simulink model "hil_fuel_cell_valve"  (R2022a)
settings: Solver=FixedStepDiscrete  StartTime=0.0  StopTime=inf  FixedStep=0.01  RelTol=1e-3  AbsTol=1e-3  EnableMultiTasking=on
model workspace: external: MATLAB File model_workspace.m (data not in the file)
values from neighbouring files (symbols this model uses):
  anode_tube_D = 0.004    [model_workspace.m]
  cathode_tube_D = 0.004    [model_workspace.m]
  env_p = 0.101325    [model_workspace.m]
  env_T = 60    [model_workspace.m]
  N2_T = [-56.55 -50 -40 -30 -20 -10 -5 -4 -3 -2 -1 0 1 2 3 4 5 10 20 30          40 50 60 70 80 90 100 110 120 130 140 150 160 170 180 190 200 210          220 230 240 250 260 270 280 290 300 310 320 330 340 350]    [model_workspace.m]
  radiator_air_area_fins = 11.5625    [model_workspace.m]
  radiator_air_area_primary = 1.2231250000000002    (= 1.223125)    [model_workspace.m]
  radiator_eta_fin = 0.7    [model_workspace.m]
  radiator_rho = 2700    [model_workspace.m]
  radiator_t_wall = 0.0001    [model_workspace.m]
  stack_area = 49    [model_workspace.m]
  stack_iL = 1.4    [model_workspace.m]
  stack_mea_rho = 1800    [model_workspace.m]
  stack_num_cells = 8    [model_workspace.m]
  stack_num_channels = 1    [model_workspace.m]
  stack_t_gdl = 250    [model_workspace.m]
  stack_t_membrane = 125    [model_workspace.m]
  stack_w_channels = 0.4    [model_workspace.m]
  time_step = 0.02    [model_workspace.m]
libraries: fl_lib x102, nesl_utility x42, simulink x7, slpidlib x3
(part 3 of 3)

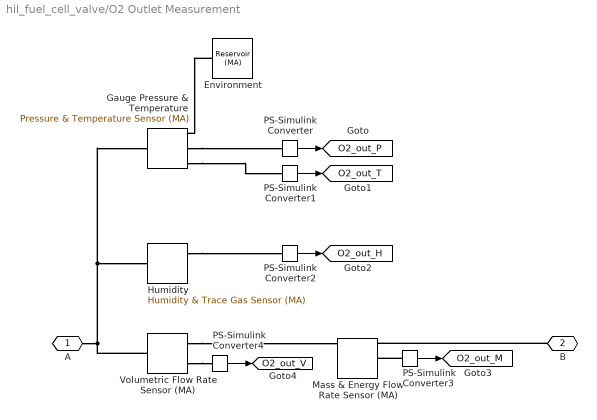
== system hil_fuel_cell_valve/O2 Outlet Measurement ==
  Environment : fl_lib/Moist Air/Elements/Reservoir (MA)  pressure_spec=foundation.enum.pressure_spec.specified  reservoir_pressure=env_p MPa  temperature_spec=foundation.enum.temperature_spec.specified  reservoir_temperature=env_T degC  moisture_spec=foundation.enum.moisture_spec.relative_humidity  reservoir_RH=0  reservoir_x_w=0.01  reservoir_y_w=0.01  reservoir_HR=0.01  trace_gas_spec=foundation.enum.trace_gas_spec.mole_fraction  reservoir_x_g=0.001  reservoir_y_g=tank_yH2  RH_ws=1  area_A=pi*anode_tube_D^2/4 m^2
      settings: SourceProductBaseCode=PW,SS,VE
  Gauge Pressure & Temperature : fl_lib/Moist Air/Sensors/Pressure & Temperature Sensor (MA)
      settings: SourceProductBaseCode=PW,SS,VE  InternalSimscapePortConfiguration="{\"Bottom\":[],\"Left\":[{\"id\":\"A\",\"label\":\"A\",\"type\":\"foundation.moist_air.moist_air\"}],\"Right\":[{\"id\":\"B\",\"label\":\"B\",\"type\":\"foundation.moist_air.moist_air\"},{\"id\":\"P\",\"label\":\"P\",\"type\":\"output\"},{\"id\":\"T\",\"label\":\"T\",\"type\":\"output\"}],\"Top\":[]}"
  Humidity : fl_lib/Moist Air/Sensors/Humidity & Trace Gas Sensor (MA)  moisture_spec=foundation.enum.moisture_spec.relative_humidity  trace_gas_spec=foundation.enum.trace_gas_spec.mass_fraction
      settings: SourceProductBaseCode=PW,SS,VE  InternalSimscapePortConfiguration="{\"Bottom\":[],\"Left\":[{\"id\":\"A\",\"label\":\"A\",\"type\":\"foundation.moist_air.moist_air\"}],\"Right\":[{\"id\":\"W\",\"label\":\"W\",\"type\":\"output\"},{\"id\":\"G\",\"label\":\"G\",\"type\":\"output\"}],\"Top\":[]}"
  Mass & Energy Flow Rate Sensor (MA) : fl_lib/Moist Air/Sensors/Mass & Energy Flow Rate Sensor (MA)
      settings: SourceProductBaseCode=PW,SS,VE  InternalSimscapePortConfiguration="{\"Bottom\":[],\"Left\":[{\"id\":\"A\",\"label\":\"A\",\"type\":\"foundation.moist_air.moist_air\"},{\"id\":\"Mw\",\"label\":\"Mw\",\"type\":\"output\"},{\"id\":\"Mg\",\"label\":\"Mg\",\"type\":\"output\"}],\"Right\":[{\"id\":\"B\",\"label\":\"B\",\"type\":\"foundation.moist_air.moist_air\"},{\"id\":\"M\",\"label\":\"M\",\"type\":\"output\"},{\"id\":\"PHI\",\"label\":\"Phi\",\"type\":\"output\"}],\"Top\":[]}"
  PS-Simulink Converter{,1..4} (5 alike) : nesl_utility/PS-Simulink Converter  PhysicalDomain=network_engine_domain  SubClassName=ps_output  LeftPortType=input  RightPortType=output  PseudoPeriodic=off  Frequencies=[]  VectorFormat=inherit  Unit=inherit  AffineConversion=off
      settings: SourceProductBaseCode=SS,PW,VE
  Volumetric Flow Rate Sensor (MA) : fl_lib/Moist Air/Sensors/Volumetric Flow Rate Sensor (MA)  volumetric_flow_conditions=foundation.enum.volumetric_flow_conditions.actual  p_std=0.101325 MPa  T_std=20 degC  RH_std=0.65
      settings: SourceProductBaseCode=PW,SS,VE  InternalSimscapePortConfiguration="{\"Bottom\":[],\"Left\":[{\"id\":\"A\",\"label\":\"A\",\"type\":\"foundation.moist_air.moist_air\"}],\"Right\":[{\"id\":\"B\",\"label\":\"B\",\"type\":\"foundation.moist_air.moist_air\"},{\"id\":\"V\",\"label\":\"V\",\"type\":\"output\"}],\"Top\":[]}"
  A : PMIOPort  Side=Left
  B : PMIOPort  Port=2  Side=Right
  tag scope: O2_out_H=global, O2_out_M=global, O2_out_P=global, O2_out_T=global, O2_out_V=global
  wires:
  PS-Simulink Converter1/1 -> [O2_out_T]
  PS-Simulink Converter2/1 -> [O2_out_H]
  PS-Simulink Converter/1 -> [O2_out_P]
  PS-Simulink Converter3/1 -> [O2_out_M]
  PS-Simulink Converter4/1 -> [O2_out_V]
  connections:
  Environment/LConn1 -- Gauge Pressure & Temperature/RConn1
  A/RConn1 -- Volumetric Flow Rate Sensor (MA)/LConn1 -- Humidity/LConn1 -- Gauge Pressure & Temperature/LConn1
  Humidity/RConn1 -- PS-Simulink Converter2/LConn1
  Gauge Pressure & Temperature/RConn3 -- PS-Simulink Converter1/LConn1
  Gauge Pressure & Temperature/RConn2 -- PS-Simulink Converter/LConn1
  PS-Simulink Converter3/LConn1 -- Mass & Energy Flow Rate Sensor (MA)/RConn2
  B/RConn1 -- Mass & Energy Flow Rate Sensor (MA)/RConn1
  Volumetric Flow Rate Sensor (MA)/RConn1 -- Mass & Energy Flow Rate Sensor (MA)/LConn1
  Volumetric Flow Rate Sensor (MA)/RConn2 -- PS-Simulink Converter4/LConn1

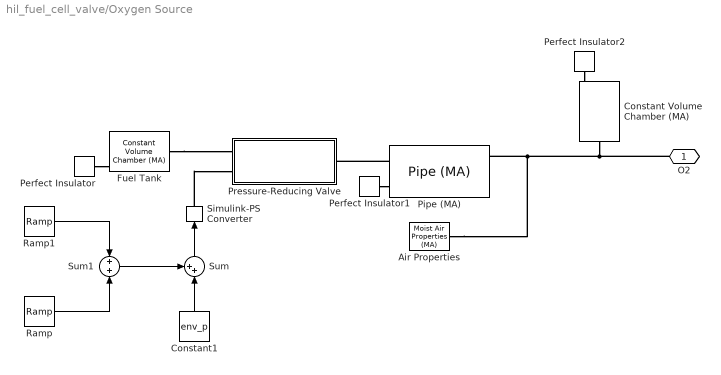
== system hil_fuel_cell_valve/Oxygen Source ==
  Air Properties : fl_lib/Moist Air/Utilities/Moist Air Properties (MA)  R_a=N2_R J/kg/K  T_TLU=N2_T degC  h_a_TLU=N2_h kJ/kg  mu_a_TLU=N2_mu s*uPa  k_a_TLU=N2_k mW/m/K  p_min=1 kPa  p_max=inf MPa  T_min=min(N2_T) degC  T_max=max(N2_T) degC  p_atm=0.101325 MPa  T_atm=20 degC  R_w=461.523 J/kg/K  p_ws_TLU=[1.71168953425982e-06; 3.93770601979424e-06; 1.28411717710344e-05; 3.80051394873809e-05; .00010323902900209; .000259873810798063; .000401741022116384; .000437454836117844; .000476040820618202; .000517704666185737; .000562664883741207; .000611212677444345; .000657088049117899; .000705987905898279; .000758082381149132; .000813549384183233; .000872574861129522; .00122818386934022; .0023392147667769; .00424668834054807; .00738442748706953; .0123512704340234; .0199458019246787; .0312006356960619; .0474147199263783; .0701823607447713; .10141797792131; .143375967241115; .198665399739302; .270259606559999; .361500961984849; .476101381081492; .618139196722055; .792053183687694; 1.0026345688121; 1.25501792086105; 1.55467186826983; 1.90739066433297; 2.31928772772542; 2.79679245576864; 3.34665187151016; 3.97593907083533; 4.69207105435535; 5.5028394740883; 6.41645928168037; 7.4416425436169; 8.58770832955728; 9.86474556030261; 11.2838558865497; 12.8575218898034; 14.6001810568052; 16.5291642526045] MPa  h_w_vap_TLU=[2836.88241275372; 2837.81392500514; 2838.63937175807; 2838.7309929628; 2838.06905313927; 2836.62597341095; 2835.60023952573; 2835.37006381376; 2835.13143158077; 2834.88429145066; 2834.62859062897; 2500.93420564316; 2498.55329907119; 2496.17495082036; 2493.79885912205; 2491.42474723191; 2489.05236104642; 2477.20875029194; 2453.54955988604; 2429.83856603313; 2406.00136954922; 2381.97406342174; 2357.69101156389; 2333.08088387814; 2308.06565480412; 2282.56034405021; 2256.47287422313; 2229.70428017508; 2202.14968030993; 2173.69998896199; 2144.24368406447; 2113.66758247452; 2081.85585110571; 2048.68725710494; 2014.03141249899; 1977.7449923284; 1939.66849592886; 1899.62342931686; 1857.40930169838; 1812.79975416601; 1765.53721731251; 1715.32525772152; 1661.81700477787; 1604.59703745016; 1543.1534616334; 1476.83692476464; 1404.80240352424; 1325.92091736114; 1238.61667822208; 1140.5102987018; 1027.62017777647; 892.733785613825] kJ/kg  h_w_TLU=[2396.55944251649; 2408.68643343608; 2427.1988031141; 2445.702165897; 2464.18429108356; 2482.62529466839; 2491.82135326629; 2493.6580151792; 2495.49372578218; 2497.32843835745; 2499.16210446923; 2500.99462758899; 2502.83092214066; 2504.6665223621; 2506.50140563013; 2508.335548891; 2510.16892865793; 2519.32352241995; 2537.56068088674; 2555.67742615292; 2573.6403223998; 2591.4109179101; 2608.9455037701; 2626.19492016262; 2643.10444358428; 2659.61377634497; 2675.58278696023; 2696.1846256545; 2716.49989553741; 2736.6235210957; 2756.61216047011; 2776.50561773853; 2796.33378922508; 2816.11979583049; 2835.88181423877; 2855.63430574511; 2875.38889327595; 2895.15500577172; 2914.94035964689; 2934.75132290228; 2954.59319330244; 2974.47041285505; 2994.38673458964; 3014.34535328009; 3034.34900867103; 3054.40006755764; 3074.50058946898; 3094.65237953784; 3114.85703128106; 3135.11596137801; 3155.43043805905; 3175.80160435813] kJ/kg  mu_w_TLU=[6.81365662228272; 7.04953750742707; 7.40970098298307; 7.76991278093907; 8.13017290129507; 8.49048134405107; 8.67065368632907; 8.70668960445667; 8.74272600580827; 8.77876289038387; 8.81480025818347; 8.85083810920707; 8.88687644345467; 8.92291526092627; 8.95895456162187; 8.99499434554147; 9.03103461268507; 9.21124319676307; 9.57169660671907; 9.93219833907507; 10.2927483938311; 10.6533467709871; 11.0139934705431; 11.3746884924991; 11.7354318368551; 12.0962235036111; 12.4570634927671; 12.8179518043231; 13.1788884382791; 13.5398733946351; 13.9009066733911; 14.2619882745471; 14.6231181981031; 14.9842964440591; 15.3455230124151; 15.7067979031711; 16.0681211163271; 16.4294926518831; 16.7909125098391; 17.1523806901951; 17.5138971929511; 17.8754620181071; 18.2370751656631; 18.5987366356191; 18.9604464279751; 19.3222045427311; 19.6840109798871; 20.0458657394431; 20.4077688213991; 20.7697202257551; 21.1317199525111; 21.4937680016671] s*uPa  k_w_TLU=[11.46288215976; 11.941997488935; 12.676358586935; 13.414208884935; 14.155548382935; 14.900377080935; 15.274099879935; 15.348949115735; 15.423833243535; 15.498752263335; 15.573706175135; 15.648694978935; 15.723718674735; 15.798777262535; 15.873870742335; 15.948999114135; 16.024162377935; 16.400502076935; 17.155798374935; 17.914583872935; 18.676858570935; 19.442622468935; 20.211875566935; 20.984617864935; 21.760849362935; 22.540570060935; 23.323779958935; 24.110479056935; 24.900667354935; 25.694344852935; 26.491511550935; 27.292167448935; 28.096312546935; 28.903946844935; 29.715070342935; 30.529683040935; 31.347784938935; 32.169376036935; 32.994456334935; 33.823025832935; 34.655084530935; 35.490632428935; 36.329669526935; 37.172195824935; 38.018211322935; 38.867716020935; 39.720709918935; 40.577193016935; 41.437165314935; 42.300626812935; 43.167577510935; 44.038017408935] mW/m/K  D_w=25 mm^2/s  trace_gas_model=foundation.enum.trace_gas_model.track_properties  R_g=O2_R J/kg/K  h_g_TLU=O2_h kJ/kg  mu_g_TLU=O2_mu s*uPa  k_g_TLU=O2_k mW/m/K  D_g=O2_D mm^2/s
      settings: SourceProductBaseCode=PW,SS,VE
      settings: AttributesFormatString=|
      | dry air --> N2
      | water vapor --> H2O
      | trace gas --> O2
  Constant Volume Chamber (MA) : fl_lib/Moist Air/Elements/Constant Volume Chamber (MA)  volume=1 l  num_ports=foundation.enum.num_ports.one  area_A=pi*anode_tube_D^2/4 m^2  area_B=0.01 m^2  area_C=0.01 m^2  area_D=0.01 m^2  RH_ws=1  time_constant=1e-3 s  moisture_trace_gas_source=foundation.enum.moisture_trace_gas_source.none  moisture_source_spec=foundation.enum.moisture_source_spec.vapor  moisture_mass_flow=0 kg/s  moisture_temperature_spec=foundation.enum.temperature_spec.atmospheric  moisture_temperature=293.15 K  trace_gas_mass_flow=0 kg/s  trace_gas_temperature_spec=foundation.enum.temperature_spec.atmospheric  trace_gas_temperature=293.15 K  p_I_specify=on  p_I_priority=High  p_I=0.101325 MPa  p_I_nominal_specify=off  p_I_nominal_unit=MPa  p_I_nominal_value=1  T_I_specify=on  T_I_priority=High  T_I=env_T degC  T_I_nominal_specify=off  T_I_nominal_unit=K  T_I_nominal_value=1  RH_I_specify=off  RH_I_priority=High  RH_I=0  RH_I_nominal_specify=off  RH_I_nominal_unit=1  RH_I_nominal_value=1  x_w_I_specify=off  x_w_I_priority=None  x_w_I=0  x_w_I_nominal_specify=off  x_w_I_nominal_unit=1  x_w_I_nominal_value=1  y_w_I_specify=off  y_w_I_priority=None  y_w_I=0  y_w_I_nominal_specify=off  y_w_I_nominal_unit=1  y_w_I_nominal_value=1  HR_I_specify=off  HR_I_priority=None  HR_I=0  HR_I_nominal_specify=off  HR_I_nominal_unit=1  HR_I_nominal_value=1  x_g_I_specify=on  x_g_I_priority=None  x_g_I=0  x_g_I_nominal_specify=off  x_g_I_nominal_unit=1  x_g_I_nominal_value=1  y_g_I_specify=on  y_g_I_priority=High  y_g_I=tank_yH2  y_g_I_nominal_specify=off  y_g_I_nominal_unit=1  y_g_I_nominal_value=1
      settings: SourceProductBaseCode=PW,SS,VE  InternalSimscapePortConfiguration="{\"Bottom\":[],\"Left\":[{\"id\":\"A\",\"label\":\"A\",\"type\":\"foundation.moist_air.moist_air\"}],\"Right\":[{\"id\":\"W\",\"label\":\"W\",\"type\":\"output\"},{\"id\":\"F\",\"label\":\"F\",\"type\":\"output\"},{\"id\":\"H\",\"label\":\"H\",\"type\":\"foundation.thermal.thermal\"}],\"Top\":[]}"
  Constant1 : Constant  Value=env_p
  Fuel Tank : fl_lib/Moist Air/Elements/Constant Volume Chamber (MA)  volume=tank_V l  num_ports=foundation.enum.num_ports.one  area_A=pi*anode_tube_D^2/4 m^2  area_B=0.01 m^2  area_C=0.01 m^2  area_D=0.01 m^2  RH_ws=1  time_constant=1e-3 s  moisture_trace_gas_source=foundation.enum.moisture_trace_gas_source.none  moisture_source_spec=foundation.enum.moisture_source_spec.vapor  moisture_mass_flow=0 kg/s  moisture_temperature_spec=foundation.enum.temperature_spec.atmospheric  moisture_temperature=293.15 K  trace_gas_mass_flow=0 kg/s  trace_gas_temperature_spec=foundation.enum.temperature_spec.atmospheric  trace_gas_temperature=293.15 K  p_I_specify=on  p_I_priority=High  p_I=tank_p MPa  p_I_nominal_specify=off  p_I_nominal_unit=MPa  p_I_nominal_value=1  T_I_specify=on  T_I_priority=High  T_I=env_T degC  T_I_nominal_specify=off  T_I_nominal_unit=K  T_I_nominal_value=1  RH_I_specify=off  RH_I_priority=High  RH_I=0  RH_I_nominal_specify=off  RH_I_nominal_unit=1  RH_I_nominal_value=1  x_w_I_specify=off  x_w_I_priority=None  x_w_I=0  x_w_I_nominal_specify=off  x_w_I_nominal_unit=1  x_w_I_nominal_value=1  y_w_I_specify=off  y_w_I_priority=None  y_w_I=0  y_w_I_nominal_specify=off  y_w_I_nominal_unit=1  y_w_I_nominal_value=1  HR_I_specify=off  HR_I_priority=None  HR_I=0  HR_I_nominal_specify=off  HR_I_nominal_unit=1  HR_I_nominal_value=1  x_g_I_specify=on  x_g_I_priority=None  x_g_I=0  x_g_I_nominal_specify=off  x_g_I_nominal_unit=1  x_g_I_nominal_value=1  y_g_I_specify=on  y_g_I_priority=High  y_g_I=tank_yH2  y_g_I_nominal_specify=off  y_g_I_nominal_unit=1  y_g_I_nominal_value=1
      settings: SourceProductBaseCode=PW,SS,VE  InternalSimscapePortConfiguration="{\"Bottom\":[],\"Left\":[{\"id\":\"A\",\"label\":\"A\",\"type\":\"foundation.moist_air.moist_air\"}],\"Right\":[{\"id\":\"W\",\"label\":\"W\",\"type\":\"output\"},{\"id\":\"F\",\"label\":\"F\",\"type\":\"output\"},{\"id\":\"H\",\"label\":\"H\",\"type\":\"foundation.thermal.thermal\"}],\"Top\":[]}"
  Perfect Insulator : fl_lib/Thermal/Thermal Elements/Perfect Insulator  T_specify=off  T_priority=None  T=0 K  T_nominal_specify=off  T_nominal_unit=K  T_nominal_value=1
      settings: SourceProductBaseCode=PW,SS,VE
  Perfect Insulator1 : fl_lib/Thermal/Thermal Elements/Perfect Insulator  T_specify=off  T_priority=None  T=0 K  T_nominal_specify=off  T_nominal_unit=K  T_nominal_value=1
      settings: SourceProductBaseCode=PW,SS,VE
  Perfect Insulator2 : fl_lib/Thermal/Thermal Elements/Perfect Insulator  T_specify=off  T_priority=None  T=0 K  T_nominal_specify=off  T_nominal_unit=K  T_nominal_value=1
      settings: SourceProductBaseCode=PW,SS,VE
  Pipe (MA) : fl_lib/Moist Air/Elements/Pipe (MA)  length=1 m  area=pi*anode_tube_D^2/4 m^2  Dh=anode_tube_D m  length_add=0.1 m  roughness=15e-6 m  Re_lam=2000  Re_tur=4000  shape_factor=64  Nu_lam=3.66  RH_ws=1  time_constant=1e-3 s  moisture_trace_gas_source=foundation.enum.moisture_trace_gas_source.none  moisture_source_spec=foundation.enum.moisture_source_spec.vapor  moisture_mass_flow=0 kg/s  moisture_temperature_spec=foundation.enum.temperature_spec.atmospheric  moisture_temperature=293.15 K  trace_gas_mass_flow=0 kg/s  trace_gas_temperature_spec=foundation.enum.temperature_spec.atmospheric  trace_gas_temperature=293.15 K  p_I_specify=on  p_I_priority=High  p_I=env_p MPa  p_I_nominal_specify=off  p_I_nominal_unit=MPa  p_I_nominal_value=1  T_I_specify=on  T_I_priority=High  T_I=env_T degC  T_I_nominal_specify=off  T_I_nominal_unit=K  T_I_nominal_value=1  RH_I_specify=off  RH_I_priority=High  RH_I=0  RH_I_nominal_specify=off  RH_I_nominal_unit=1  RH_I_nominal_value=1  x_w_I_specify=off  x_w_I_priority=None  x_w_I=0  x_w_I_nominal_specify=off  x_w_I_nominal_unit=1  x_w_I_nominal_value=1  y_w_I_specify=off  y_w_I_priority=None  y_w_I=0  y_w_I_nominal_specify=off  y_w_I_nominal_unit=1  y_w_I_nominal_value=1  HR_I_specify=off  HR_I_priority=None  HR_I=0  HR_I_nominal_specify=off  HR_I_nominal_unit=1  HR_I_nominal_value=1  x_g_I_specify=on  x_g_I_priority=None  x_g_I=0  x_g_I_nominal_specify=off  x_g_I_nominal_unit=1  x_g_I_nominal_value=1  y_g_I_specify=on  y_g_I_priority=High  y_g_I=tank_yH2  y_g_I_nominal_specify=off  y_g_I_nominal_unit=1  y_g_I_nominal_value=1
      settings: SourceProductBaseCode=PW,SS,VE
  Pressure-Reducing Valve : Subsystem  Tag=PublishSubsystem  mask(Pressure-Reducing Valve){D=anode_tube_D, r_min=1e-4, r_max=0.2, p_range=0.005}
      mask prompts: D "Connecting tube diameter (m)"; r_min "Min diameter ratio"; r_max "Max diameter ratio"; p_range "Pressure regulation range (MPa)"
      mask help: This subsystem models a pressure reducing valve that maintains a set pressure at port B. The valve is normally open. When the pressure is above the set pressure, it is fully closed.
  Ramp : simulink/Sources/Ramp  slope=0.001  start=0.5  InitialOutput=0.2
  Ramp1 : simulink/Sources/Ramp  slope=-0.001  start=5  InitialOutput=0
  Simulink-PS Converter : nesl_utility/Simulink-PS Converter  PhysicalDomain=network_engine_domain  SubClassName=ps_input  LeftPortType=input  RightPortType=output  PseudoPeriodic=off  Frequencies=[]  NoiseDistribution=none  NoiseParameters=[]  Unit=MPa  AffineConversion=off  FilteringAndDerivatives=provide  SimscapeFilterOrder=1  InputFilterTimeConstant=0.001  UdotUserProvided=0
      settings: SourceProductBaseCode=SS,PW,VE
  Sum : Sum  Inputs=++|
  Sum1 : Sum  Inputs=+|+
  O2 : PMIOPort  Side=Right
  wires:
  Sum/1 -> Simulink-PS Converter/1
  Constant1/1 -> Sum/2
  Sum1/1 -> Sum/1
  Ramp/1 -> Sum1/2
  Ramp1/1 -> Sum1/1
  connections:
  Perfect Insulator1/LConn1 -- Pipe (MA)/LConn2
  O2/RConn1 -- Constant Volume Chamber (MA)/LConn1 -- Air Properties/RConn1 -- Pipe (MA)/RConn1
  Pipe (MA)/LConn1 -- Pressure-Reducing Valve/RConn1
  Simulink-PS Converter/RConn1 -- Pressure-Reducing Valve/LConn2
  Fuel Tank/LConn1 -- Pressure-Reducing Valve/LConn1
  Perfect Insulator/LConn1 -- Fuel Tank/RConn3
  Perfect Insulator2/LConn1 -- Constant Volume Chamber (MA)/RConn3

== system hil_fuel_cell_valve/Pressure Measurements ==
  note: In this block the pressure measurements are converted from Pa to bar.
  Gain{,1..3} (4 alike) : Gain  Gain=1e-5
  H2in : Outport
  H2out : Outport  Port=2
  O2in : Outport  Port=3
  O2out : Outport  Port=4
  wires:
  [H2_in_P] -> Gain/1
  [O2_out_P] -> Gain3/1
  [H2_out_P] -> Gain1/1
  [O2_in_P] -> Gain2/1
  Gain/1 -> H2in/1
  Gain1/1 -> H2out/1
  Gain2/1 -> O2in/1
  Gain3/1 -> O2out/1

== system hil_fuel_cell_valve/Temperature Measurements ==
  H2in : Outport
  H2out : Outport  Port=2
  O2in : Outport  Port=3
  O2out : Outport  Port=4
  wires:
  [H2_out_T] -> H2out/1
  [O2_in_T] -> O2in/1
  [H2_in_T] -> H2in/1
  [O2_out_T] -> O2out/1

== system hil_fuel_cell_valve/Volumetric Flow Measurements ==
  note: In this block the mass flow rate has a unit of m^3/s.
  H2in : Outport
  H2out : Outport  Port=2
  O2in : Outport  Port=3
  O2out : Outport  Port=4
  wires:
  [H2_in_V] -> H2in/1
  [H2_out_V] -> H2out/1
  [O2_in_V] -> O2in/1
  [O2_out_V] -> O2out/1

== system hil_fuel_cell_valve/Anode Exhaust/Pressure Relief Valve ==
  Absolute Reference (MA) : fl_lib/Moist Air/Elements/Absolute Reference (MA)
      settings: SourceProductBaseCode=PW,SS,VE
  PS Add : fl_lib/Physical Signals/Functions/PS Add
      settings: SourceProductBaseCode=PW,SS,VE
  PS Constant : fl_lib/Physical Signals/Sources/PS Constant  constant=r_min^2
      settings: SourceProductBaseCode=PW,SS,VE
  PS Gain : fl_lib/Physical Signals/Functions/PS Gain  gain=(r_max^2 - r_min^2)/p_range 1/MPa
      settings: SourceProductBaseCode=PW,SS,VE
  PS Gain1 : fl_lib/Physical Signals/Functions/PS Gain  gain=pi*D^2/4 m^2
      settings: SourceProductBaseCode=PW,SS,VE
  PS Subtract : fl_lib/Physical Signals/Functions/PS Subtract
      settings: SourceProductBaseCode=PW,SS,VE
  Pressure & Temperature Sensor (MA) : fl_lib/Moist Air/Sensors/Pressure & Temperature Sensor (MA)
      settings: SourceProductBaseCode=PW,SS,VE  InternalSimscapePortConfiguration="{\"Bottom\":[],\"Left\":[{\"id\":\"A\",\"label\":\"A\",\"type\":\"foundation.moist_air.moist_air\"}],\"Right\":[{\"id\":\"B\",\"label\":\"B\",\"type\":\"foundation.moist_air.moist_air\"},{\"id\":\"P\",\"label\":\"P\",\"type\":\"output\"},{\"id\":\"T\",\"label\":\"T\",\"type\":\"output\"}],\"Top\":[]}"
  Valve : fl_lib/Moist Air/Elements/Local Restriction (MA)  restriction_type=foundation.enum.restriction_type.variable  restriction_area=0.001 m^2  min_area=pi*(r_min*D)^2/4 m^2  max_area=pi*(r_max*D)^2/4 m^2  area=pi*D^2/4 m^2  Cd=0.64  B_lam=0.999
      settings: SourceProductBaseCode=PW,SS,VE
  A : PMIOPort  Side=Left
  B : PMIOPort  Port=2  Side=Right
  p_set : PMIOPort  Port=3  Side=Left
  connections:
  PS Add/RConn1 -- PS Gain1/LConn1
  PS Gain/LConn1 -- PS Subtract/RConn1
  PS Gain1/RConn1 -- Valve/LConn2
  Absolute Reference (MA)/LConn1 -- Pressure & Temperature Sensor (MA)/RConn1
  Valve/RConn1 -- B/RConn1
  Valve/LConn1 -- A/RConn1 -- Pressure & Temperature Sensor (MA)/LConn1
  PS Gain/RConn1 -- PS Add/LConn1
  PS Add/LConn2 -- PS Constant/RConn1
  Pressure & Temperature Sensor (MA)/RConn2 -- PS Subtract/LConn1
  p_set/RConn1 -- PS Subtract/LConn2

== system hil_fuel_cell_valve/Cathode Exhaust/Pressure Relief Valve ==
  Absolute Reference (MA) : fl_lib/Moist Air/Elements/Absolute Reference (MA)
      settings: SourceProductBaseCode=PW,SS,VE
  PS Add : fl_lib/Physical Signals/Functions/PS Add
      settings: SourceProductBaseCode=PW,SS,VE
  PS Constant : fl_lib/Physical Signals/Sources/PS Constant  constant=r_min^2
      settings: SourceProductBaseCode=PW,SS,VE
  PS Gain : fl_lib/Physical Signals/Functions/PS Gain  gain=(r_max^2 - r_min^2)/p_range 1/MPa
      settings: SourceProductBaseCode=PW,SS,VE
  PS Gain1 : fl_lib/Physical Signals/Functions/PS Gain  gain=pi*D^2/4 m^2
      settings: SourceProductBaseCode=PW,SS,VE
  PS Subtract : fl_lib/Physical Signals/Functions/PS Subtract
      settings: SourceProductBaseCode=PW,SS,VE
  Pressure & Temperature Sensor (MA) : fl_lib/Moist Air/Sensors/Pressure & Temperature Sensor (MA)
      settings: SourceProductBaseCode=PW,SS,VE  InternalSimscapePortConfiguration="{\"Bottom\":[],\"Left\":[{\"id\":\"A\",\"label\":\"A\",\"type\":\"foundation.moist_air.moist_air\"}],\"Right\":[{\"id\":\"B\",\"label\":\"B\",\"type\":\"foundation.moist_air.moist_air\"},{\"id\":\"P\",\"label\":\"P\",\"type\":\"output\"},{\"id\":\"T\",\"label\":\"T\",\"type\":\"output\"}],\"Top\":[]}"
  Valve : fl_lib/Moist Air/Elements/Local Restriction (MA)  restriction_type=foundation.enum.restriction_type.variable  restriction_area=0.001 m^2  min_area=pi*(r_min*D)^2/4 m^2  max_area=pi*(r_max*D)^2/4 m^2  area=pi*D^2/4 m^2  Cd=0.64  B_lam=0.999
      settings: SourceProductBaseCode=PW,SS,VE
  A : PMIOPort  Side=Left
  B : PMIOPort  Port=2  Side=Right
  p_set : PMIOPort  Port=3  Side=Left
  connections:
  PS Add/RConn1 -- PS Gain1/LConn1
  PS Gain/LConn1 -- PS Subtract/RConn1
  PS Gain1/RConn1 -- Valve/LConn2
  Absolute Reference (MA)/LConn1 -- Pressure & Temperature Sensor (MA)/RConn1
  Valve/RConn1 -- B/RConn1
  Valve/LConn1 -- A/RConn1 -- Pressure & Temperature Sensor (MA)/LConn1
  PS Gain/RConn1 -- PS Add/LConn1
  PS Add/LConn2 -- PS Constant/RConn1
  Pressure & Temperature Sensor (MA)/RConn2 -- PS Subtract/LConn1
  p_set/RConn1 -- PS Subtract/LConn2

== system hil_fuel_cell_valve/Control Unit/Anode Humidifier Control ==
  H2_in_H : Inport
  Proportional Control : Subsystem
      settings: PortSchema="{\"entries\":[{\"content\":{\"sides\":[{\"content\":{\"connectorIds\":[\"Out1\"]},\"type\":\"ConnectorPlacement.EquallySpacedRectSide\",\"uuid\":\"33b0bb19-6ca8-4c2f-a8e5-38c79e2d4ea7\"},{\"content\":{\"connectorIds\":[\"In1\",\"In2\"],\"side\":\"RIGHT\"},\"type\":\"ConnectorPlacement.EquallySpacedRectSide\",\"uuid\":\"2d3d0fb5-30df-4063-9961-aa14a50037fc\"},{\"content\":{\"connectorIds\":[],\"side\":\"TOP\"},\"type\":\"ConnectorPlacement.EquallySpacedRectSide\",\"uuid\":\"001eb165-7a82-4caa-be7c-fe6eb836d372\"}]},\"type\":\"ConnectorPlacement.EquallySpacedConnector\",\"uuid\":\"bcf88336-5c7e-4fc8-879e-8d7ff57e5e5f\"}],\"packageUris\":[\"http://schema.mathworks.com/mf0/Connector/R2020b\"],\"version\":\"1.0\"}"
  Relative Humidity : Constant
  H2_cl_H : Outport
  wires:
  Proportional Control/1(Mw) -> H2_cl_H/1
  H2_in_H/1 -> Proportional Control/2(RH_meas)
  Relative Humidity/1 -> Proportional Control/1(RH_set)

== system hil_fuel_cell_valve/Control Unit/Cathode Humidifier Control ==
  O2_in_H : Inport
  Proportional Control : Subsystem
  Relative Humidity : Constant
  O2_cl_H : Outport
  wires:
  O2_in_H/1 -> Proportional Control/2(RH_meas)
  Relative Humidity/1 -> Proportional Control/1(RH_set)
  Proportional Control/1(Mw) -> O2_cl_H/1

== system hil_fuel_cell_valve/Control Unit/Coolant Pump Control ==
  C_in_T : Inport
  Pump Control : Subsystem
  Stack Temperature : Constant  Value=80
  C_cl_T : Outport
  wires:
  Stack Temperature/1 -> Pump Control/1(T_set)
  C_in_T/1 -> Pump Control/2(T_meas)
  Pump Control/1(cmd) -> C_cl_T/1

== system hil_fuel_cell_valve/Control Unit/Hydrogen Recirculation Control ==
  L_on_i : Inport
  Feedforward Control : Subsystem
  H2_cl_H2 : Outport
  wires:
  L_on_i/1 -> Feedforward Control/1(i)
  Feedforward Control/1(cmd) -> H2_cl_H2/1

== system hil_fuel_cell_valve/Control Unit/Subsystem ==
  L_on_i : Inport
  O2_in_M : Inport  Port=2
  Compressor Control : Subsystem
  Oxygen Excess Ratio : Constant  Value=2.5
  O2_cl_O2 : Outport
  wires:
  L_on_i/1 -> Compressor Control/2(i)
  Oxygen Excess Ratio/1 -> Compressor Control/1(OER)
  Compressor Control/1(cmd) -> O2_cl_O2/1
  O2_in_M/1 -> Compressor Control/3(M_meas)

== system hil_fuel_cell_valve/Electrical Load/Inputs ==
  Drive Cycle Power Demand : Subsystem  VariantControl=Drive cycle
      settings: PortSchema="{\"entries\":[{\"content\":{\"sides\":[{\"content\":{\"connectorIds\":[\"LConn1\"]},\"type\":\"ConnectorPlacement.EquallySpacedRectSide\",\"uuid\":\"316ab41f-9548-4c29-941b-82cd3006a9cc\"},{\"content\":{\"connectorIds\":[],\"side\":\"RIGHT\"},\"type\":\"ConnectorPlacement.EquallySpacedRectSide\",\"uuid\":\"21ddf6a1-5f8a-47a4-ab15-3c27c3a556ce\"},{\"content\":{\"connectorIds\":[\"LConn2\"],\"side\":\"TOP\"},\"type\":\"ConnectorPlacement.EquallySpacedRectSide\",\"uuid\":\"59191a52-f145-4ac2-9cf2-0e0b54b3d2a8\"}]},\"type\":\"ConnectorPlacement.EquallySpacedConnector\",\"uuid\":\"e8f988fd-b412-4b1a-aaea-374cf82170cc\"}],\"packageUris\":[\"http://schema.mathworks.com/mf0/Connector/R2020b\"],\"version\":\"1.0\"}"
      mask Display:
      | plot(0, 0)
      | plot(100, 100)
      | 
      | mws = get_param(bdroot, 'ModelWorkspace');
      | x = getVariable(mws, 'drive_cycle_time');
      | y = getVariable(mws, 'drive_cycle_power');
      | 
      | plot(x/max(x)*80 + 10, y/max(y)*60 + 30)
  Ramp Current Demand : Subsystem  VariantControl=Ramp
      settings: PortSchema="{\"entries\":[{\"content\":{\"sides\":[{\"content\":{\"connectorIds\":[\"LConn1\"]},\"type\":\"ConnectorPlacement.EquallySpacedRectSide\",\"uuid\":\"316ab41f-9548-4c29-941b-82cd3006a9cc\"},{\"content\":{\"connectorIds\":[],\"side\":\"RIGHT\"},\"type\":\"ConnectorPlacement.EquallySpacedRectSide\",\"uuid\":\"21ddf6a1-5f8a-47a4-ab15-3c27c3a556ce\"},{\"content\":{\"connectorIds\":[\"LConn2\"],\"side\":\"TOP\"},\"type\":\"ConnectorPlacement.EquallySpacedRectSide\",\"uuid\":\"59191a52-f145-4ac2-9cf2-0e0b54b3d2a8\"}]},\"type\":\"ConnectorPlacement.EquallySpacedConnector\",\"uuid\":\"e8f988fd-b412-4b1a-aaea-374cf82170cc\"}],\"packageUris\":[\"http://schema.mathworks.com/mf0/Connector/R2020b\"],\"version\":\"1.0\"}"
      mask Display:
      | plot(0, 0)
      | plot(100, 100)
      | 
      | plot([20 40 80], [20 20 90])
  Ramped Step Current Demand : Subsystem  VariantControl=Ramped Step
      settings: PortSchema="{\"entries\":[{\"content\":{\"sides\":[{\"content\":{\"connectorIds\":[\"LConn1\"]},\"type\":\"ConnectorPlacement.EquallySpacedRectSide\",\"uuid\":\"316ab41f-9548-4c29-941b-82cd3006a9cc\"},{\"content\":{\"connectorIds\":[],\"side\":\"RIGHT\"},\"type\":\"ConnectorPlacement.EquallySpacedRectSide\",\"uuid\":\"21ddf6a1-5f8a-47a4-ab15-3c27c3a556ce\"},{\"content\":{\"connectorIds\":[\"LConn2\"],\"side\":\"TOP\"},\"type\":\"ConnectorPlacement.EquallySpacedRectSide\",\"uuid\":\"59191a52-f145-4ac2-9cf2-0e0b54b3d2a8\"}]},\"type\":\"ConnectorPlacement.EquallySpacedConnector\",\"uuid\":\"e8f988fd-b412-4b1a-aaea-374cf82170cc\"}],\"packageUris\":[\"http://schema.mathworks.com/mf0/Connector/R2020b\"],\"version\":\"1.0\"}"
      mask Display:
      | plot(0, 0)
      | plot(100, 100)
      | 
      | plot([20 40 60 80], [20 20 80 80])
  Step Current Demand : Subsystem  VariantControl=Step
      settings: PortSchema="{\"entries\":[{\"content\":{\"sides\":[{\"content\":{\"connectorIds\":[\"LConn1\"]},\"type\":\"ConnectorPlacement.EquallySpacedRectSide\",\"uuid\":\"316ab41f-9548-4c29-941b-82cd3006a9cc\"},{\"content\":{\"connectorIds\":[],\"side\":\"RIGHT\"},\"type\":\"ConnectorPlacement.EquallySpacedRectSide\",\"uuid\":\"21ddf6a1-5f8a-47a4-ab15-3c27c3a556ce\"},{\"content\":{\"connectorIds\":[\"LConn2\"],\"side\":\"TOP\"},\"type\":\"ConnectorPlacement.EquallySpacedRectSide\",\"uuid\":\"59191a52-f145-4ac2-9cf2-0e0b54b3d2a8\"}]},\"type\":\"ConnectorPlacement.EquallySpacedConnector\",\"uuid\":\"e8f988fd-b412-4b1a-aaea-374cf82170cc\"}],\"packageUris\":[\"http://schema.mathworks.com/mf0/Connector/R2020b\"],\"version\":\"1.0\"}"
      mask Display:
      | plot(0, 0)
      | plot(100, 100)
      | 
      | plot([20 50 50 80], [20 20 80 80])
  i : PMIOPort  Side=Left
  v : PMIOPort  Port=2  Side=Left

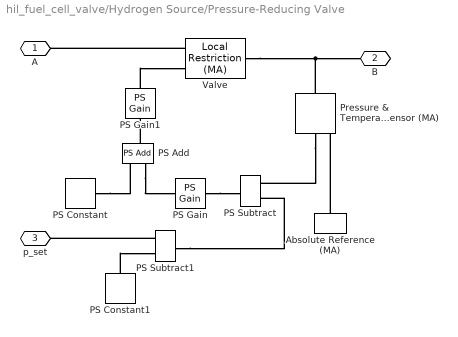
== system hil_fuel_cell_valve/Hydrogen Source/Pressure-Reducing Valve ==
  Absolute Reference (MA) : fl_lib/Moist Air/Elements/Absolute Reference (MA)
      settings: SourceProductBaseCode=PW,SS,VE
  PS Add : fl_lib/Physical Signals/Functions/PS Add
      settings: SourceProductBaseCode=PW,SS,VE
  PS Constant : fl_lib/Physical Signals/Sources/PS Constant  constant=r_max^2
      settings: SourceProductBaseCode=PW,SS,VE
  PS Constant1 : fl_lib/Physical Signals/Sources/PS Constant  constant=p_range MPa
      settings: SourceProductBaseCode=PW,SS,VE
  PS Gain : fl_lib/Physical Signals/Functions/PS Gain  gain=(r_min^2 - r_max^2)/p_range 1/MPa
      settings: SourceProductBaseCode=PW,SS,VE
  PS Gain1 : fl_lib/Physical Signals/Functions/PS Gain  gain=pi*D^2/4 m^2
      settings: SourceProductBaseCode=PW,SS,VE
  PS Subtract : fl_lib/Physical Signals/Functions/PS Subtract
      settings: SourceProductBaseCode=PW,SS,VE
  PS Subtract1 : fl_lib/Physical Signals/Functions/PS Subtract
      settings: SourceProductBaseCode=PW,SS,VE
  Pressure & Temperature Sensor (MA) : fl_lib/Moist Air/Sensors/Pressure & Temperature Sensor (MA)
      settings: SourceProductBaseCode=PW,SS,VE  InternalSimscapePortConfiguration="{\"Bottom\":[],\"Left\":[{\"id\":\"A\",\"label\":\"A\",\"type\":\"foundation.moist_air.moist_air\"}],\"Right\":[{\"id\":\"B\",\"label\":\"B\",\"type\":\"foundation.moist_air.moist_air\"},{\"id\":\"P\",\"label\":\"P\",\"type\":\"output\"},{\"id\":\"T\",\"label\":\"T\",\"type\":\"output\"}],\"Top\":[]}"
  Valve : fl_lib/Moist Air/Elements/Local Restriction (MA)  restriction_type=foundation.enum.restriction_type.variable  restriction_area=0.001 m^2  min_area=pi*(r_min*D)^2/4 m^2  max_area=pi*(r_max*D)^2/4 m^2  area=pi*D^2/4 m^2  Cd=0.64  B_lam=0.999
      settings: SourceProductBaseCode=PW,SS,VE
  A : PMIOPort  Side=Left
  B : PMIOPort  Port=2  Side=Right
  p_set : PMIOPort  Port=3  Side=Left
  connections:
  PS Constant1/RConn1 -- PS Subtract1/LConn2
  PS Subtract1/LConn1 -- p_set/RConn1
  PS Subtract1/RConn1 -- PS Subtract/LConn2
  PS Constant/RConn1 -- PS Add/LConn1
  PS Add/LConn2 -- PS Gain/RConn1
  PS Add/RConn1 -- PS Gain1/LConn1
  PS Gain/LConn1 -- PS Subtract/RConn1
  Pressure & Temperature Sensor (MA)/RConn2 -- PS Subtract/LConn1
  PS Gain1/RConn1 -- Valve/LConn2
  Absolute Reference (MA)/LConn1 -- Pressure & Temperature Sensor (MA)/RConn1
  Pressure & Temperature Sensor (MA)/LConn1 -- B/RConn1 -- Valve/RConn1
  Valve/LConn1 -- A/RConn1

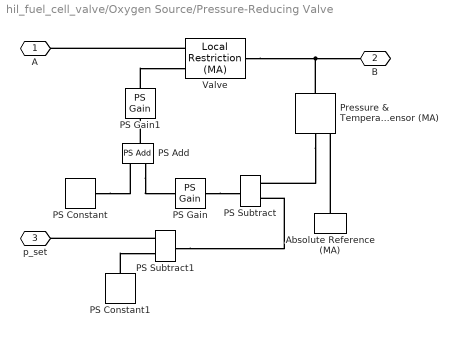
== system hil_fuel_cell_valve/Oxygen Source/Pressure-Reducing Valve ==
  Absolute Reference (MA) : fl_lib/Moist Air/Elements/Absolute Reference (MA)
      settings: SourceProductBaseCode=PW,SS,VE
  PS Add : fl_lib/Physical Signals/Functions/PS Add
      settings: SourceProductBaseCode=PW,SS,VE
  PS Constant : fl_lib/Physical Signals/Sources/PS Constant  constant=r_max^2
      settings: SourceProductBaseCode=PW,SS,VE
  PS Constant1 : fl_lib/Physical Signals/Sources/PS Constant  constant=p_range MPa
      settings: SourceProductBaseCode=PW,SS,VE
  PS Gain : fl_lib/Physical Signals/Functions/PS Gain  gain=(r_min^2 - r_max^2)/p_range 1/MPa
      settings: SourceProductBaseCode=PW,SS,VE
  PS Gain1 : fl_lib/Physical Signals/Functions/PS Gain  gain=pi*D^2/4 m^2
      settings: SourceProductBaseCode=PW,SS,VE
  PS Subtract : fl_lib/Physical Signals/Functions/PS Subtract
      settings: SourceProductBaseCode=PW,SS,VE
  PS Subtract1 : fl_lib/Physical Signals/Functions/PS Subtract
      settings: SourceProductBaseCode=PW,SS,VE
  Pressure & Temperature Sensor (MA) : fl_lib/Moist Air/Sensors/Pressure & Temperature Sensor (MA)
      settings: SourceProductBaseCode=PW,SS,VE  InternalSimscapePortConfiguration="{\"Bottom\":[],\"Left\":[{\"id\":\"A\",\"label\":\"A\",\"type\":\"foundation.moist_air.moist_air\"}],\"Right\":[{\"id\":\"B\",\"label\":\"B\",\"type\":\"foundation.moist_air.moist_air\"},{\"id\":\"P\",\"label\":\"P\",\"type\":\"output\"},{\"id\":\"T\",\"label\":\"T\",\"type\":\"output\"}],\"Top\":[]}"
  Valve : fl_lib/Moist Air/Elements/Local Restriction (MA)  restriction_type=foundation.enum.restriction_type.variable  restriction_area=0.001 m^2  min_area=pi*(r_min*D)^2/4 m^2  max_area=pi*(r_max*D)^2/4 m^2  area=pi*D^2/4 m^2  Cd=0.64  B_lam=0.999
      settings: SourceProductBaseCode=PW,SS,VE
  A : PMIOPort  Side=Left
  B : PMIOPort  Port=2  Side=Right
  p_set : PMIOPort  Port=3  Side=Left
  connections:
  PS Constant1/RConn1 -- PS Subtract1/LConn2
  PS Subtract1/LConn1 -- p_set/RConn1
  PS Subtract1/RConn1 -- PS Subtract/LConn2
  PS Constant/RConn1 -- PS Add/LConn1
  PS Add/LConn2 -- PS Gain/RConn1
  PS Add/RConn1 -- PS Gain1/LConn1
  PS Gain/LConn1 -- PS Subtract/RConn1
  Pressure & Temperature Sensor (MA)/RConn2 -- PS Subtract/LConn1
  PS Gain1/RConn1 -- Valve/LConn2
  Absolute Reference (MA)/LConn1 -- Pressure & Temperature Sensor (MA)/RConn1
  Pressure & Temperature Sensor (MA)/LConn1 -- B/RConn1 -- Valve/RConn1
  Valve/LConn1 -- A/RConn1

== system hil_fuel_cell_valve/Control Unit/Anode Humidifier Control/Proportional Control ==
  RH_set : Inport
  RH_meas : Inport  Port=2
  Gain : Gain  Gain=0.001
  Sum : Sum  Inputs=|+-
  Mw : Outport
  wires:
  RH_meas/1 -> Sum/2
  RH_set/1 -> Sum/1
  Sum/1 -> Gain/1
  Gain/1 -> Mw/1

== system hil_fuel_cell_valve/Control Unit/Cathode Humidifier Control/Proportional Control ==
  RH_set : Inport
  RH_meas : Inport  Port=2
  Gain : Gain  Gain=0.001
  Sum : Sum  Inputs=|+-
  Mw : Outport
  wires:
  RH_meas/1 -> Sum/2
  Sum/1 -> Gain/1
  RH_set/1 -> Sum/1
  Gain/1 -> Mw/1

== system hil_fuel_cell_valve/Control Unit/Coolant Pump Control/Pump Control ==
  T_set : Inport
  T_meas : Inport  Port=2
  Control Signals : Scope  NumInputPorts=2
  Mux : Mux  Inputs=2
  Mux1 : Mux  Inputs=2
  PID Controller : slpidlib/PID Controller  Controller=PI  Form=Ideal  TimeDomain=Discrete-time  UseExternalTs=off  SampleTime=-1  IntegratorMethod=Forward Euler  FilterMethod=Forward Euler  ControllerParametersSource=internal  P=0.100000000000000  I=0.010000000000000  UseKiTs=off  D=0.000000000000000  N=78.693868057473310  UseFilter=on  TunerSelectOption=Transfer Function Based (PID Tuner App)  ZeroCross=off  InitialConditionSource=internal  InitialConditionForIntegrator=0  InitialConditionForFilter=0  DifferentiatorICPrevScaledInput=0  ExternalReset=none  TrackingMode=off  Kt=1  LimitOutput=on  SatLimitsSource=internal  UpperSaturationLimit=1  LowerSaturationLimit=0  LinearizeAsGain=on  AntiWindupMode=clamping  Kb=1  POutMin=[]  POutMax=[]  IOutMin=[]  IOutMax=[]  DOutMin=[]  DOutMax=[]  NOutMin=[]  NOutMax=[]  SumOutMin=[]  SumOutMax=[]  SaturationOutMin=[]  SaturationOutMax=[]  PParamMin=[]  PParamMax=[]  IParamMin=[]  IParamMax=[]  DParamMin=[]  DParamMax=[]  NParamMin=[]  NParamMax=[]  KbParamMin=[]  KbParamMax=[]  KtParamMin=[]  KtParamMax=[]  KbOutMin=[]  KbOutMax=[]  KtOutMin=[]  KtOutMax=[]  IntegratorOutMin=[]  IntegratorOutMax=[]  FilterOutMin=[]  FilterOutMax=[]  SumI1OutMin=[]  SumI1OutMax=[]  SumI2OutMin=[]  SumI2OutMax=[]  SumI3OutMin=[]  SumI3OutMax=[]  SumI4OutMin=[]  SumI4OutMax=[]  SumDOutMin=[]  SumDOutMax=[]  DifferentiatorOutMin=[]  DifferentiatorOutMax=[]  FilterDiffOutCoefMin=[]  FilterDiffOutCoefMax=[]  ReciprocalOutMin=[]  ReciprocalOutMax=[]  SumDenOutMin=[]  SumDenOutMax=[]  SumNumOutMin=[]  SumNumOutMax=[]  DivideOutMin=[]  DivideOutMax=[]  UdiffTsProdOutMin=[]  UdiffTsProdOutMax=[]  NTsProdOutMin=[]  NTsProdOutMax=[]  UintegralTsProdOutMin=[]  UintegralTsProdOutMax=[]  UngainTsProdOutMin=[]  UngainTsProdOutMax=[]  IntegratorContinuousStateAttributes=''  IntegratorStateMustResolveToSignalObject=off  IntegratorRTWStateStorageClass=Auto  FilterContinuousStateAttributes=''  FilterStateMustResolveToSignalObject=off  FilterRTWStateStorageClass=Auto  ParallelPVariant=Passthrough  IdealPVariant=InternalParameters  IVariant=InternalParameters  DVariant=Disabled  IntegratorVariant=Discrete  SatVariant=Enabled  AWVariant=DiscClampingIdeal  PCopyVariant=InternalParamsIdeal  TRVariant=Disabled  FdbkBlocksVariant=Forward  IdealPFdbkVariant=Disabled  SatFdbkVariant=Disabled  DerivativeFilterVariant=Disabled  NVariant=Disabled  NCopyVariant=Disabled_SignalSpec  FilterICVariant=Disabled  IntegratorICVariant=InternalICs  ExternalResetVariant=Disabled  TRSumVariant=Passthrough  SumFdbkVariant=Disabled  SumVariant=Sum_PI  TsampFilterVariant=InternalTs  TsampNgainVariant=Passthrough  TsampIntegralVariant=Passthrough  ExternalSaturationOutDataTypeStr=Inherit: Same as second input  aMode=0
  Sum : Sum  Inputs=|-+
  cmd : Outport
  wires:
  PID Controller/1 -> Mux1/2, cmd/1, Mux1/1
  T_set/1 -> Mux/1, Sum/1
  T_meas/1 -> Mux/2, Sum/2
  Sum/1 -> PID Controller/1
  Mux/1 -> Control Signals/1
  Mux1/1 -> Control Signals/2

== system hil_fuel_cell_valve/Control Unit/Hydrogen Recirculation Control/Feedforward Control ==
  i : Inport
  Constant : Constant  Value=0.2
  Gain : Gain  Gain=0.8 / (stack_iL * stack_area)
  Saturation : Saturate  UpperLimit=1  LowerLimit=0  ZeroCross=off
  Sum : Sum  Inputs=|++
  cmd : Outport
  wires:
  i/1 -> Gain/1
  Saturation/1 -> cmd/1
  Gain/1 -> Sum/1
  Constant/1 -> Sum/2
  Sum/1 -> Saturation/1

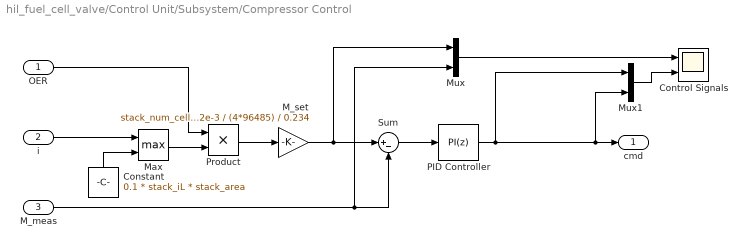
== system hil_fuel_cell_valve/Control Unit/Subsystem/Compressor Control ==
  OER : Inport
  i : Inport  Port=2
  M_meas : Inport  Port=3
  Constant : Constant  Value=0.1 * stack_iL * stack_area
  Control Signals : Scope  NumInputPorts=2
  M_set : Gain  Gain=stack_num_cells * 32e-3 / (4*96485) / 0.234
  Max : MinMax  Function=max  Inputs=2  ZeroCross=off
  Mux : Mux  Inputs=2
  Mux1 : Mux  Inputs=2
  PID Controller : slpidlib/PID Controller  Controller=PI  Form=Ideal  TimeDomain=Discrete-time  UseExternalTs=off  SampleTime=-1  IntegratorMethod=Forward Euler  FilterMethod=Forward Euler  ControllerParametersSource=internal  P=5.000000000000000  I=0.500000000000000  UseKiTs=off  D=0.000000000000000  N=78.693868057473310  UseFilter=on  TunerSelectOption=Transfer Function Based (PID Tuner App)  ZeroCross=off  InitialConditionSource=internal  InitialConditionForIntegrator=0  InitialConditionForFilter=0  DifferentiatorICPrevScaledInput=0  ExternalReset=none  TrackingMode=off  Kt=1  LimitOutput=on  SatLimitsSource=internal  UpperSaturationLimit=1  LowerSaturationLimit=0  LinearizeAsGain=on  AntiWindupMode=clamping  Kb=1  POutMin=[]  POutMax=[]  IOutMin=[]  IOutMax=[]  DOutMin=[]  DOutMax=[]  NOutMin=[]  NOutMax=[]  SumOutMin=[]  SumOutMax=[]  SaturationOutMin=[]  SaturationOutMax=[]  PParamMin=[]  PParamMax=[]  IParamMin=[]  IParamMax=[]  DParamMin=[]  DParamMax=[]  NParamMin=[]  NParamMax=[]  KbParamMin=[]  KbParamMax=[]  KtParamMin=[]  KtParamMax=[]  KbOutMin=[]  KbOutMax=[]  KtOutMin=[]  KtOutMax=[]  IntegratorOutMin=[]  IntegratorOutMax=[]  FilterOutMin=[]  FilterOutMax=[]  SumI1OutMin=[]  SumI1OutMax=[]  SumI2OutMin=[]  SumI2OutMax=[]  SumI3OutMin=[]  SumI3OutMax=[]  SumI4OutMin=[]  SumI4OutMax=[]  SumDOutMin=[]  SumDOutMax=[]  DifferentiatorOutMin=[]  DifferentiatorOutMax=[]  FilterDiffOutCoefMin=[]  FilterDiffOutCoefMax=[]  ReciprocalOutMin=[]  ReciprocalOutMax=[]  SumDenOutMin=[]  SumDenOutMax=[]  SumNumOutMin=[]  SumNumOutMax=[]  DivideOutMin=[]  DivideOutMax=[]  UdiffTsProdOutMin=[]  UdiffTsProdOutMax=[]  NTsProdOutMin=[]  NTsProdOutMax=[]  UintegralTsProdOutMin=[]  UintegralTsProdOutMax=[]  UngainTsProdOutMin=[]  UngainTsProdOutMax=[]  IntegratorContinuousStateAttributes=''  IntegratorStateMustResolveToSignalObject=off  IntegratorRTWStateStorageClass=Auto  FilterContinuousStateAttributes=''  FilterStateMustResolveToSignalObject=off  FilterRTWStateStorageClass=Auto  ParallelPVariant=Passthrough  IdealPVariant=InternalParameters  IVariant=InternalParameters  DVariant=Disabled  IntegratorVariant=Discrete  SatVariant=Enabled  AWVariant=DiscClampingIdeal  PCopyVariant=InternalParamsIdeal  TRVariant=Disabled  FdbkBlocksVariant=Forward  IdealPFdbkVariant=Disabled  SatFdbkVariant=Disabled  DerivativeFilterVariant=Disabled  NVariant=Disabled  NCopyVariant=Disabled_SignalSpec  FilterICVariant=Disabled  IntegratorICVariant=InternalICs  ExternalResetVariant=Disabled  TRSumVariant=Passthrough  SumFdbkVariant=Disabled  SumVariant=Sum_PI  TsampFilterVariant=InternalTs  TsampNgainVariant=Passthrough  TsampIntegralVariant=Passthrough  ExternalSaturationOutDataTypeStr=Inherit: Same as second input  aMode=0
  Product : Product
  Sum : Sum  Inputs=|+-
  cmd : Outport
  wires:
  OER/1 -> Product/1
  Constant/1 -> Max/2
  i/1 -> Max/1
  Max/1 -> Product/2
  Sum/1 -> PID Controller/1
  M_set/1 -> Sum/1, Mux/1
  Product/1 -> M_set/1
  M_meas/1 -> Mux/2, Sum/2
  PID Controller/1 -> Mux1/2, cmd/1, Mux1/1
  Mux/1 -> Control Signals/1
  Mux1/1 -> Control Signals/2

== system hil_fuel_cell_valve/Electrical Load/Inputs/Drive Cycle Power Demand ==
  From Workspace : FromWorkspace  VariableName=[drive_cycle_time, drive_cycle_power]
  PS Divide : fl_lib/Physical Signals/Functions/PS Divide
      settings: SourceProductBaseCode=PW,SS,VE
  PS-Simulink Converter : nesl_utility/PS-Simulink Converter  PhysicalDomain=network_engine_domain  SubClassName=ps_output  LeftPortType=input  RightPortType=output  PseudoPeriodic=off  Frequencies=[]  VectorFormat=1-D array  Unit=V  AffineConversion=off
      settings: SourceProductBaseCode=SS,PW,VE
  PS-Simulink Converter1 : nesl_utility/PS-Simulink Converter  PhysicalDomain=network_engine_domain  SubClassName=ps_output  LeftPortType=input  RightPortType=output  PseudoPeriodic=off  Frequencies=[]  VectorFormat=1-D array  Unit=A  AffineConversion=off
      settings: SourceProductBaseCode=SS,PW,VE
  Simulink-PS Converter : nesl_utility/Simulink-PS Converter  PhysicalDomain=network_engine_domain  SubClassName=ps_input  LeftPortType=input  RightPortType=output  PseudoPeriodic=off  Frequencies=[]  NoiseDistribution=none  NoiseParameters=[]  Unit=kW  AffineConversion=off  FilteringAndDerivatives=provide  SimscapeFilterOrder=1  InputFilterTimeConstant=0.001  UdotUserProvided=0
      settings: SourceProductBaseCode=SS,PW,VE
  i : PMIOPort  Side=Left
  v : PMIOPort  Port=2  Side=Left
  tag scope: i_stack=global, v_stack=global
  wires:
  From Workspace/1 -> Simulink-PS Converter/1
  PS-Simulink Converter/1 -> [v_stack]
  PS-Simulink Converter1/1 -> [i_stack]
  connections:
  PS Divide/LConn1 -- Simulink-PS Converter/RConn1
  i/RConn1 -- PS Divide/RConn1 -- PS-Simulink Converter1/LConn1
  v/RConn1 -- PS-Simulink Converter/LConn1 -- PS Divide/LConn2

== system hil_fuel_cell_valve/Electrical Load/Inputs/Ramp Current Demand ==
  PS-Simulink Converter : nesl_utility/PS-Simulink Converter  PhysicalDomain=network_engine_domain  SubClassName=ps_output  LeftPortType=input  RightPortType=output  PseudoPeriodic=off  Frequencies=[]  VectorFormat=1-D array  Unit=V  AffineConversion=off
      settings: SourceProductBaseCode=SS,PW,VE
  Ramp : simulink/Sources/Ramp  slope=stack_iL * stack_area * (1 - 1e-6) / (2500 - 100)  start=5  InitialOutput=0
  Simulink-PS Converter : nesl_utility/Simulink-PS Converter  PhysicalDomain=network_engine_domain  SubClassName=ps_input  LeftPortType=input  RightPortType=output  PseudoPeriodic=off  Frequencies=[]  NoiseDistribution=none  NoiseParameters=[]  Unit=A  AffineConversion=off  FilteringAndDerivatives=provide  SimscapeFilterOrder=1  InputFilterTimeConstant=0.001  UdotUserProvided=0
      settings: SourceProductBaseCode=SS,PW,VE
  i : PMIOPort  Side=Left
  v : PMIOPort  Port=2  Side=Left
  tag scope: i_stack=global, v_stack=global
  wires:
  Ramp/1 -> Simulink-PS Converter/1, [i_stack]
  PS-Simulink Converter/1 -> [v_stack]
  connections:
  Simulink-PS Converter/RConn1 -- i/RConn1
  v/RConn1 -- PS-Simulink Converter/LConn1

== system hil_fuel_cell_valve/Electrical Load/Inputs/Ramped Step Current Demand ==
  PS-Simulink Converter : nesl_utility/PS-Simulink Converter  PhysicalDomain=network_engine_domain  SubClassName=ps_output  LeftPortType=input  RightPortType=output  PseudoPeriodic=off  Frequencies=[]  VectorFormat=1-D array  Unit=V  AffineConversion=off
      settings: SourceProductBaseCode=SS,PW,VE
  Ramp : simulink/Sources/Ramp  slope=stack_iL * stack_area * (1 - 1e-6) / (2500 - 100)  start=5  InitialOutput=0
  Ramp1 : simulink/Sources/Ramp  slope=- stack_iL * stack_area * (1 - 1e-6) / (2500 - 100)  start=15  InitialOutput=0
  Simulink-PS Converter : nesl_utility/Simulink-PS Converter  PhysicalDomain=network_engine_domain  SubClassName=ps_input  LeftPortType=input  RightPortType=output  PseudoPeriodic=off  Frequencies=[]  NoiseDistribution=none  NoiseParameters=[]  Unit=A  AffineConversion=off  FilteringAndDerivatives=provide  SimscapeFilterOrder=1  InputFilterTimeConstant=0.001  UdotUserProvided=0
      settings: SourceProductBaseCode=SS,PW,VE
  Sum : Sum  Inputs=+|+
  i : PMIOPort  Side=Left
  v : PMIOPort  Port=2  Side=Left
  tag scope: i_stack=global, v_stack=global
  wires:
  PS-Simulink Converter/1 -> [v_stack]
  Sum/1 -> [i_stack], Simulink-PS Converter/1
  Ramp/1 -> Sum/1
  Ramp1/1 -> Sum/2
  connections:
  Simulink-PS Converter/RConn1 -- i/RConn1
  v/RConn1 -- PS-Simulink Converter/LConn1

== system hil_fuel_cell_valve/Electrical Load/Inputs/Step Current Demand ==
  PS-Simulink Converter : nesl_utility/PS-Simulink Converter  PhysicalDomain=network_engine_domain  SubClassName=ps_output  LeftPortType=input  RightPortType=output  PseudoPeriodic=off  Frequencies=[]  VectorFormat=1-D array  Unit=V  AffineConversion=off
      settings: SourceProductBaseCode=SS,PW,VE
  Simulink-PS Converter : nesl_utility/Simulink-PS Converter  PhysicalDomain=network_engine_domain  SubClassName=ps_input  LeftPortType=input  RightPortType=output  PseudoPeriodic=off  Frequencies=[]  NoiseDistribution=none  NoiseParameters=[]  Unit=A  AffineConversion=off  FilteringAndDerivatives=provide  SimscapeFilterOrder=1  InputFilterTimeConstant=0.001  UdotUserProvided=0
      settings: SourceProductBaseCode=SS,PW,VE
  Step : Step  Time=5  After=0.5 * stack_iL * stack_area  SampleTime=0
  i : PMIOPort  Side=Left
  v : PMIOPort  Port=2  Side=Left
  tag scope: i_stack=global, v_stack=global
  wires:
  Step/1 -> [i_stack], Simulink-PS Converter/1
  PS-Simulink Converter/1 -> [v_stack]
  connections:
  Simulink-PS Converter/RConn1 -- i/RConn1
  PS-Simulink Converter/LConn1 -- v/RConn1
